simulink model "PassVeh7DOF"  (R2024b)
settings: Solver=ode14x  StartTime=0.0  StopTime=30  FixedStep=0.001  RelTol=1e-1
model workspace (MAT data in the model file):
  A_mu = 10
  B_reff = 8.386
  CONVERTER_DATA = [0 0.1 0.2 0.3 0.4 0.5 0.6 0.7 0.8 0.81 0.82 0.83 ... (63 elements, 21x3)]
  Cps = 2
  Cz = 7766.25
  DOWN_TABLE = [0 0 0 0 0 0 5 5 7.5 7.5 15 15 ... (30 elements, 6x5)]
  DOWN_TH_BP = [0 5 40 50 90 100]
  D_reff = 0.25826
  EMAP = [-40 215 245 264 264 267 267 267 267 267 -44 117 ... (110 elements, 10x11)]
  F0z = [6086.4 4324.8]
  F_reff = 0.07394
  F_zmax = 10000
  F_zmin = 100
  F_zo = 4000
  Kz = 48000
  MF : object (value not decoded)
  NCyl = 6
  NE_VEC = [800 1200 1600 2000 2400 2800 3200 3600 4000 4400 4800]
  Pstd = 101325
  R_eff = 0.298
  Rair = 287
  SUS : object (value not decoded)
  TH_VEC = [0; 20; 30; 40; 50; 60; 70; 80; 90; 100]
  TWAITdn = 1.25
  TWAITup = 0.1
  Tin = [1 2 3 4 5 6 7 8 9 10 2 2 ... (20 elements, 10x2)]
  Tstd = 293.15
  UP_TABLE = [7.5 7.5 15 25 40 40 25 25 35 45 70 80 ... (30 elements, 6x5)]
  UP_TH_BP = [0 25 35 50 90 100]
  VEH : object (value not decoded)
  V_o = 16.7
  V_xlow = 1
  Vd = 0.00346
  WH : object (value not decoded)
  a = 1.515
  alpha_max = 1.5
  alpha_min = -1.5
  b = 1.504
  c_zo = 209651
  epsilon = 0.1
  f_air = [0 0 0 0 0 0 0 0 0 0 0 0 ... (256 elements, 16x16)]
  f_co = [0 0 0 0 0 0 0 0 0 0 0 0 ... (256 elements, 16x16)]
  f_co2 = [0 0 0 0 0 0 0 0 0 0 0 0 ... (256 elements, 16x16)]
  f_eff = [352.135682859 352.135682859 320.724378192 303.655312657 295.930136708 291.240087194 291.240271258 291.240312459 291.240275452 291.240198499 291.240100781 291.240018769 ... (256 elements, 16x16)]
  f_fuel = [0 0 0 0 0 0 0 0 0 0 0 0 ... (256 elements, 16x16)]
  f_hc = [0 0 0 0 0 0 0 0 0 0 0 0 ... (256 elements, 16x16)]
  f_nox = [0 0 0 0 0 0 0 0 0 0 0 0 ... (256 elements, 16x16)]
  f_pm = [0 0 0 0 0 0 0 0 0 0 0 0 ... (256 elements, 16x16)]
  f_susp_axl_bp = [1 2]
  f_susp_dz_bp = [-4 -0.14 -0.13 -0.12 -0.11 -0.1 -0.09 -0.08 -0.07 -0.06 -0.05 -0.04 ... (31 elements, 1x31)]
  f_susp_dzdot_bp = [-4 -0.14 -0.13 -0.12 -0.11 -0.1 -0.09 -0.08 -0.07 -0.06 -0.05 -0.04 ... (31 elements, 1x31)]
  f_susp_fmz = [-213379.591456 -28099.591456 -27619.591456 -27139.591456 -26659.591456 -26179.591456 -25699.591456 -25219.591456 -24739.591456 -24259.591456 -23779.591456 -23299.591456 ... (468968 elements, 31x31x61x2x4)]
  f_susp_geom = [-0.832564012244 0.043269987756 0.045538987756 0.047807987756 0.050076987756 0.052345987756 0.054614987756 0.056883987756 0.059152987756 0.061421987756 0.063690987756 0.065959987756 ... (11346 elements, 31x61x2x3)]
  f_susp_strgdelta_bp = [-0.523598775598 -0.506145483078 -0.488692190558 -0.471238898038 -0.453785605519 -0.436332312999 -0.418879020479 -0.401425727959 -0.383972435439 -0.366519142919 -0.349065850399 -0.331612557879 ... (61 elements, 1x61)]
  f_tbrake = [0 76.8593923996 105.140482948 131.533638111 157.926793274 176.658631717 176.65727296 176.656856686 176.656879077 176.657093756 176.657404516 176.65772406 ... (256 elements, 16x16)]
  f_tbrake_n_bpt = [0 649.519052838 912.419621844 1175.32019085 1438.22075986 1701.12132886 1964.02189787 2226.92246687 2489.82303588 2752.72360489 3015.62417389 3278.5247429 ... (16 elements, 1x16)]
  f_tbrake_t_bpt = [0 34.6410161514 61.0341713143 87.4273264773 113.82048164 140.213636803 166.606791966 192.999947129 219.393102292 245.786257455 272.179412618 298.572567781 ... (16 elements, 1x16)]
  f_texh = [766.752464599 766.752464599 786.17542386 801.679939032 884.591982581 910.574397722 910.571871054 910.570774534 910.570601632 910.570821151 910.571247242 910.571639815 ... (256 elements, 16x16)]
  f_twc_eff_co = [0.17 0.25 0.45 0.99 0.99 0.99 0.99]
  f_twc_eff_hc = [0.21 0.375 0.75 0.98 0.98 0.98 0.98]
  f_twc_eff_lam = [0.909090909 0.944055944 0.979020979 1 1.013986014 1.048951049 1.083916084]
  f_twc_eff_nox = [0.98 0.98 0.98 0.97 0.05 0.02 0]
  h = 0.134
  k_z = 50
  kappa_max = 1.5
  kappa_min = -1.5
  lam_Cx = 1
  lam_Cy = 1
  lam_Cz = 1
  lam_Ex = 1
  lam_Ey = 1
  lam_F_zo = 1
  lam_Hx = 1
  lam_Hy = 1
  lam_Kxkappa = 1
  lam_Kyalpha = 1
  lam_Kygamma = 1
  lam_Kzgamma = 1
  lam_Mr = 1
  lam_Mx = 1
  lam_My = 1
  lam_S = 1
  lam_VMx = 1
  lam_Vx = 1
  lam_Vy = 1
  lam_Vykappa = 1
  lam_muV = 0
  lam_mux = 1
  lam_muy = 1
  lam_t = 1
  lam_xalpha = 1
  lam_ykappa = 1
  numWheel = 4
  p_Cx1 = 1.579
  p_Cy1 = 1.3332
  p_Dx1 = 1.0422
  p_Dx2 = -0.08285
  p_Dx3 = 0
  p_Dy1 = 0.8784
  p_Dy2 = -0.06445
  p_Dy3 = 0
  p_Ex1 = 0.11185
  p_Ex2 = 0.3127
  p_Ex3 = 0
  p_Ex4 = 0.001603
  p_Ey1 = -0.8227
  p_Ey2 = -0.6062
  p_Ey3 = 0.09825
  p_Ey4 = -6.546
  p_Ey5 = 0
  p_Fz1 = 0.7098
  p_Hx1 = 0.00021585
  p_Hx2 = 0.0011538
  p_Hy1 = -0.0018043
  p_Hy2 = 0.003518
  p_Kx1 = 21.69
  p_Kx2 = 13.774
  p_Kx3 = -0.4119
  p_Ky1 = -15.314
  p_Ky2 = 1.7044
  p_Ky3 = 0.36986
  p_Ky4 = 1.9896
  p_Ky5 = 0
  p_Ky6 = -0.9004
  p_Ky7 = -0.2328
  p_Vx1 = 1.5973e-05
  p_Vx2 = 0.0001043
  p_Vy1 = -0.006642
  p_Vy2 = 0.03597
  p_Vy3 = -0.1621
  p_Vy4 = -0.4908
  p_pmx1 = 0
  p_px1 = -0.3489
  p_px2 = 0.382
  p_px3 = -0.09634
  p_px4 = 0.06447
  p_py1 = -0.6249
  p_py2 = -0.06535
  p_py3 = -0.1668
  p_py4 = 0.2834
  p_py5 = 0
  path : object (value not decoded)
  pio = 220000
  q_Fcx = 0
  q_Fz2 = 15.4
  q_Fzy = 0
  q_reo = 0.9974
  q_sx1 = -0.007764
  q_sx10 = 0.2824
  q_sx11 = 5.349
  q_sx12 = 0
  q_sx13 = 0
  q_sx14 = 0
  q_sx2 = 1.1915
  q_sx3 = 0.013948
  q_sx4 = 4.912
  q_sx5 = 1.02
  q_sx6 = 22.83
  q_sx7 = 0.7104
  q_sx8 = -0.023393
  q_sx9 = 0.6581
  q_sy1 = 0.00702
  q_sy2 = 0
  q_sy3 = 0.001515
  q_sy4 = 8.514e-05
  q_sy5 = 0
  q_sy6 = 0
  q_sy7 = 0.9008
  q_sy8 = -0.4089
  q_v1 = 0.0007742
  q_v2 = 0.04667
  r_Bx1 = 12.531
  r_Bx2 = 9.532
  r_Bx3 = 0
  r_By1 = 10.615
  r_By2 = 7.705
  r_By3 = 3.433e-06
  r_By4 = 0
  r_Cx1 = 1.019
  r_Cy1 = 1.0585
  r_Ex1 = -0.4487
  r_Ex2 = -0.4726
  r_Ey1 = 0.3132
  r_Ey2 = 7.63e-06
  r_Hx1 = 0.0002374
  r_Hy1 = 0.011646
  r_Hy2 = 7.63e-06
  r_Vy1 = 0.05654
  r_Vy2 = 7.63e-06
  r_Vy3 = 0
  r_Vy4 = 99.9
  r_Vy5 = 2
  r_Vy6 = 15.814
  r_o = 0.3135
  reqTmaxT = [nan 0.285774810084 0.647179872268 nan nan nan nan nan nan nan nan nan ... (168 elements, 21x8)]
  vehSpd = [0 2.77777777778 5.55555555556 8.33333333333 11.1111111111 13.8888888889 16.6666666667 19.4444444444 22.2222222222 25 27.7777777778 30.5555555556 ... (21 elements, 1x21)]
  vehWidth = 2
  w = 1
symbols that are objects in the model workspace (value not decoded): VEH
undefined symbols (not defined in the file or in its folder): Fzz, Fzzdot, InertFrm, pFz, psi, vdyntiremask, x_o, zdotFz, zFz
libraries: simulink x4, sharedTrackingLibrary x1, mcbcontrolslib x1
(part 6 of 24)

== system PassVeh7DOF/Longitudinal Wheels 4DOF/Veh2Tire/Wheel to Body Transform ==
  VelVeh : Inport  Partition=on  PartitionDimension=2  PartitionWidth=1  PartitionOffset=0
  WhlAng : Inport  Port=2  Partition=on  PartitionDimension=2  PartitionWidth=1  PartitionOffset=0
  Demux1 : Demux  Outputs=3
  Divide1 : Product  Inputs=**  Multiplication=Matrix(*)
  For Each : ForEach  DisableCoverage=on
  Rotation Angles to Direction Cosine Matrix : Subsystem  mask(Ang2DCM){rotationOrder=ZYX, aMode=2}
      mask prompts: rotationOrder "shared_aeroblks:sharedaeroblktransform:blockAng2DCMParamRotationOrder"
      mask help: shared_aeroblks:sharedaeroblktransform:blockAng2DCMDesc
      mask init:
      | if aerosharedtest(gcb)
      |     ports=aerosharedicon('sharedang2dcm');
      | else
      |     ports=sharedautoicon('sharedang2dcm');
      | end
      settings: AttributesFormatString=Rotation Order: %<rotationOrder>
      mask Help: eval('if license(''test'',''Aerospace_Blockset'')aerosharedhelp(''rotation_angles_to_direction_cosine_matrix'');elseif license(''test'',''Powertrain_Blockset'')sharedautohelp(''rotation_angles_to_direction_cosine_matrix'');end')
      mask TypeOptions rotationOrder: shared_aeroblks:sharedaeroblktransform:blockParamComboZYX | shared_aeroblks:sharedaeroblktransform:blockParamComboZYZ | shared_aeroblks:sharedaeroblktransform:blockParamComboZXY | shared_aeroblks:sharedaeroblktransform:blockParamComboZXZ | shared_aeroblks:sharedaeroblktransform:blockParamComboYXZ | shared_aeroblks:sharedaeroblktransform:blockParamComboYXY | shared_aeroblks:sharedaeroblktransform:blockParamComboYZX | shared_aeroblks:sharedaeroblktransform:blockParamComboYZY | shared_aeroblks:sharedaeroblktransform:blockParamComboXYZ | shared_aeroblks:sharedaeroblktransform:blockParamComboXYX | shared_aeroblks:sharedaeroblktransform:blockParamComboXZY | shared_aeroblks:sharedaeroblktransform:blockParamComboXZX
      mask DialogControl rotationOrder Prompt: Rotation order:
      mask Display:
      | port_label('input',1,'[R_1,R_2,R_3]','texmode','on')
      | port_label('output',1,'DCM_{be}','texmode','on')
  Selector : Selector  InputPortWidth=3  IndexOptions=Index vector (dialog)  Indices=[3 2 1]  OutputSizes=1
  xdotWheel : Outport  ConcatenationDimension=1  VectorParamsAs1DForOutWhenUnconnected=off
  ydotWheel : Outport  Port=2  ConcatenationDimension=1  VectorParamsAs1DForOutWhenUnconnected=off
  zdotWheel : Outport  Port=3  ConcatenationDimension=1  VectorParamsAs1DForOutWhenUnconnected=off
  wires:
  Divide1/1 -> Demux1/1
  Demux1/1 -> xdotWheel/1
  Demux1/2 -> ydotWheel/1
  Demux1/3 -> zdotWheel/1
  Rotation Angles to Direction Cosine Matrix/1(Out1) -> Divide1/1
  VelVeh/1 -> Divide1/2
  WhlAng/1 -> Selector/1
  Selector/1 -> Rotation Angles to Direction Cosine Matrix/1(In1)

== system PassVeh7DOF/Longitudinal Wheels 4DOF/Velocity and Vertical Load/Bicycle ==
  VehFdbk : Inport
  Bicycle Fz : Subsystem
  Bicycle V : Subsystem
  VehVel : Outport  PortDimensions=[3,4]  VectorParamsAs1DForOutWhenUnconnected=off
  Fz : Outport  Port=2  VectorParamsAs1DForOutWhenUnconnected=off
  wires:
  VehFdbk/1 -> Bicycle V/1(In1), Bicycle Fz/1(VehFdbk)
  Bicycle V/1(Out1) -> VehVel/1
  Bicycle Fz/1(Out1) -> Fz/1

== system PassVeh7DOF/Longitudinal Wheels 4DOF/Velocity and Vertical Load/Dual ==
  VehFdbk : Inport
  Dual Fz : Subsystem
  Dual V : Subsystem
  VehVel : Outport  VectorParamsAs1DForOutWhenUnconnected=off
  Fz : Outport  Port=2  VectorParamsAs1DForOutWhenUnconnected=off
  wires:
  Dual V/1(Out1) -> VehVel/1
  VehFdbk/1 -> Dual Fz/1(In1), Dual V/1(In1)
  Dual Fz/1(Out1) -> Fz/1

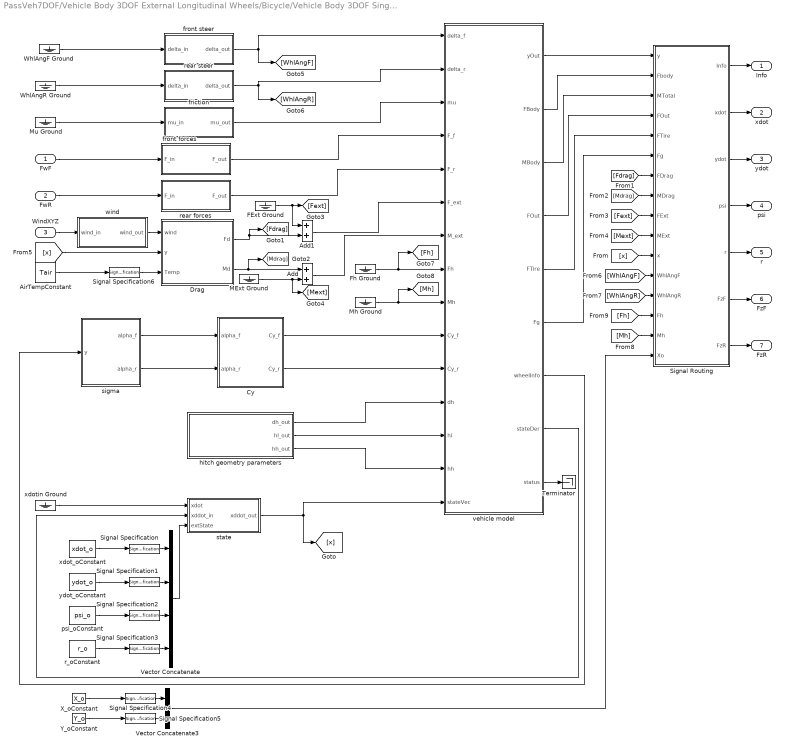
== system PassVeh7DOF/Vehicle Body 3DOF External Longitudinal Wheels/Bicycle/Vehicle Body 3DOF Single Track ==
  FwF : Inport
  FwR : Inport  Port=2
  WindXYZ : Inport  Port=3
  Add : Sum
  Add1 : Sum
  AirTempConstant : Constant  Value=Tair
  Cy : Subsystem  Variant=on  VariantControlMode=label  LabelModeActiveChoice=0
  Drag : Subsystem
  FExt Ground : Ground
  Fh Ground : Ground
  MExt Ground : Ground
  Mh Ground : Ground
  Mu Ground : Ground
  Signal Routing : Subsystem  Variant=on  VariantControlMode=label  LabelModeActiveChoice=0
  Signal Specification : SignalSpecification  Unit=m/s
  Signal Specification1 : SignalSpecification  Unit=m/s
  Signal Specification2 : SignalSpecification  Unit=rad
  Signal Specification3 : SignalSpecification  Unit=rad/s
  Signal Specification4 : SignalSpecification  Unit=m
  Signal Specification5 : SignalSpecification  Unit=m
  Signal Specification6 : SignalSpecification  Unit=K
  Terminator : Terminator
  Vector Concatenate : Concatenate  NumInputs=4
  Vector Concatenate3 : Concatenate
  WhlAngF Ground : Ground
  WhlAngR Ground : Ground
  X_oConstant : Constant  Value=X_o
  Y_oConstant : Constant  Value=Y_o
  friction : Subsystem  Variant=on  VariantControlMode=label  LabelModeActiveChoice=0
  front forces : Subsystem  Variant=on  VariantControlMode=label  LabelModeActiveChoice=2
  front steer : Subsystem  Variant=on  VariantControlMode=label  LabelModeActiveChoice=0
  hitch geometry parameters : Subsystem  Variant=on  VariantControlMode=label  LabelModeActiveChoice=3
  psi_oConstant : Constant  Value=psi_o
  r_oConstant : Constant  Value=r_o
  rear forces : Subsystem  Variant=on  VariantControlMode=label  LabelModeActiveChoice=2
  rear steer : Subsystem  Variant=on  VariantControlMode=label  LabelModeActiveChoice=0
  sigma : Subsystem  Variant=on  VariantControlMode=label  LabelModeActiveChoice=0
  state : Subsystem  Variant=on  VariantControlMode=label  LabelModeActiveChoice=0
  vehicle model : MATLAB Function  TreatAsAtomicUnit=on
  wind : Subsystem  Variant=on  VariantControlMode=label  LabelModeActiveChoice=1
  xdot_oConstant : Constant  Value=xdot_o
  xdotin Ground : Ground
  ydot_oConstant : Constant  Value=ydot_o
  Info : Outport  VectorParamsAs1DForOutWhenUnconnected=off
  xdot : Outport  Port=2  VectorParamsAs1DForOutWhenUnconnected=off
  ydot : Outport  Port=3  VectorParamsAs1DForOutWhenUnconnected=off
  psi : Outport  Port=4  VectorParamsAs1DForOutWhenUnconnected=off
  r : Outport  Port=5  VectorParamsAs1DForOutWhenUnconnected=off
  FzF : Outport  Port=6  VectorParamsAs1DForOutWhenUnconnected=off
  FzR : Outport  Port=7  VectorParamsAs1DForOutWhenUnconnected=off
  wires:
  AirTempConstant/1 -> Signal Specification6/1
  [Fh] -> Signal Routing/14(Fh)
  [Mh] -> Signal Routing/15(Mh)
  hitch geometry parameters/3(hh_out) -> vehicle model/14(hh)
  hitch geometry parameters/2(hl_out) -> vehicle model/13(hl)
  hitch geometry parameters/1(dh_out) -> vehicle model/12(dh)
  Mh Ground/1 -> [Mh], vehicle model/9(Mh)
  Fh Ground/1 -> [Fh], vehicle model/8(Fh)
  FExt Ground/1 -> [Fext], Add1/1
  MExt Ground/1 -> Add/2, [Mext]
  FwR/1 -> rear forces/1(F_in)
  FwF/1 -> front forces/1(F_in)
  xdotin Ground/1 -> state/1(xdot)
  Signal Specification6/1 -> Drag/3(Temp)
  Signal Specification5/1 -> Vector Concatenate3/2
  Y_oConstant/1 -> Signal Specification5/1
  Signal Specification4/1 -> Vector Concatenate3/1
  X_oConstant/1 -> Signal Specification4/1
  Vector Concatenate3/1 -> Signal Routing/16(Xo)
  Signal Specification2/1 -> Vector Concatenate/3
  Signal Specification3/1 -> Vector Concatenate/4
  psi_oConstant/1 -> Signal Specification2/1
  r_oConstant/1 -> Signal Specification3/1
  Signal Specification1/1 -> Vector Concatenate/2
  ydot_oConstant/1 -> Signal Specification1/1
  Signal Specification/1 -> Vector Concatenate/1
  xdot_oConstant/1 -> Signal Specification/1
  Vector Concatenate/1 -> state/3(extState)
  [WhlAngR] -> Signal Routing/13(WhlAngR)
  [WhlAngF] -> Signal Routing/12(WhlAngF)
  Signal Routing/4(psi) -> psi/1
  Mu Ground/1 -> friction/1(mu_in)
  WhlAngR Ground/1 -> rear steer/1(delta_in)
  [x] -> Drag/2(y)
  Drag/1(Fd) -> [Fdrag], Add1/2
  wind/1(wind_out) -> Drag/1(wind)
  Drag/2(Md) -> Add/1, [Mdrag]
  rear forces/1(F_out) -> vehicle model/5(F_r)
  front forces/1(F_out) -> vehicle model/4(F_f)
  vehicle model/7(wheelInfo) -> sigma/1(y)
  Signal Routing/1(Info) -> Info/1
  sigma/2(alpha_r) -> Cy/2(alpha_r)
  sigma/1(alpha_f) -> Cy/1(alpha_f)
  rear steer/1(delta_out) -> vehicle model/2(delta_r), [WhlAngR]
  front steer/1(delta_out) -> vehicle model/1(delta_f), [WhlAngF]
  Cy/2(Cy_r) -> vehicle model/11(Cy_r)
  Cy/1(Cy_f) -> vehicle model/10(Cy_f)
  friction/1(mu_out) -> vehicle model/3(mu)
  vehicle model/8(stateDer) -> state/2(xddot_in)
  vehicle model/1(yOut) -> Signal Routing/1(y)
  Signal Routing/3(ydot) -> ydot/1
  Signal Routing/5(r) -> r/1
  Signal Routing/6(FzF) -> FzF/1
  Signal Routing/7(FzR) -> FzR/1
  Signal Routing/2(xdot) -> xdot/1
  vehicle model/4(FOut) -> Signal Routing/4(FOut)
  state/1(xddot_out) -> vehicle model/15(stateVec), [x]
  [x] -> Signal Routing/11(x)
  vehicle model/9(status) -> Terminator/1
  vehicle model/5(FTire) -> Signal Routing/5(FTire)
  vehicle model/6(Fg) -> Signal Routing/6(Fg)
  [Fext] -> Signal Routing/9(FExt)
  [Fdrag] -> Signal Routing/7(FDrag)
  [Mdrag] -> Signal Routing/8(MDrag)
  [Mext] -> Signal Routing/10(MExt)
  vehicle model/2(FBody) -> Signal Routing/2(Fbody)
  vehicle model/3(MBody) -> Signal Routing/3(MTotal)
  Add/1 -> vehicle model/7(M_ext)
  Add1/1 -> vehicle model/6(F_ext)
  WhlAngF Ground/1 -> front steer/1(delta_in)
  WindXYZ/1 -> wind/1(wind_in)

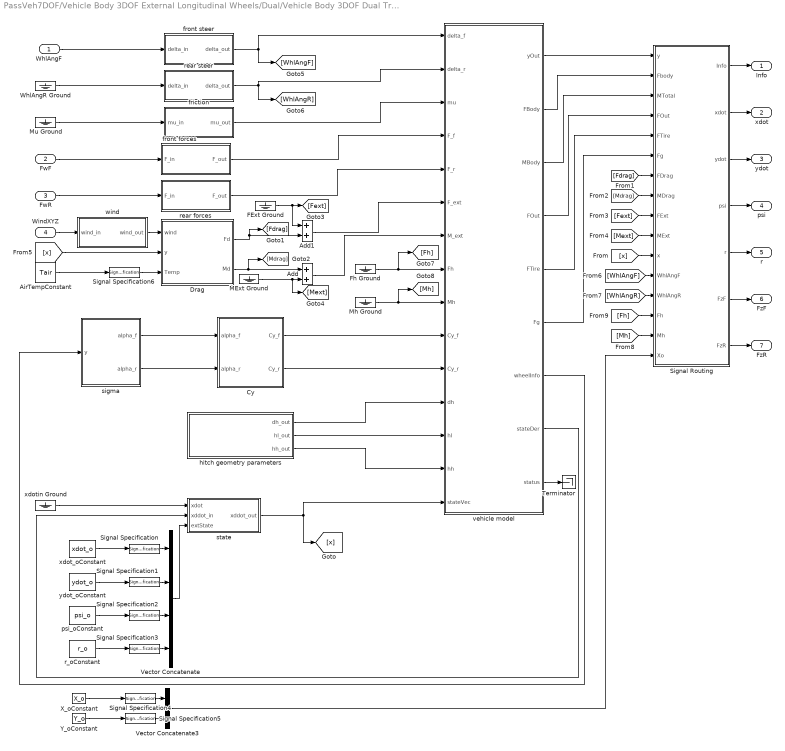
== system PassVeh7DOF/Vehicle Body 3DOF External Longitudinal Wheels/Dual/Vehicle Body 3DOF Dual Track ==
  WhlAngF : Inport
  FwF : Inport  Port=2
  FwR : Inport  Port=3
  WindXYZ : Inport  Port=4
  Add : Sum
  Add1 : Sum
  AirTempConstant : Constant  Value=Tair
  Cy : Subsystem  Variant=on  VariantControlMode=label  LabelModeActiveChoice=2
  Drag : Subsystem
  FExt Ground : Ground
  Fh Ground : Ground
  MExt Ground : Ground
  Mh Ground : Ground
  Mu Ground : Ground
  Signal Routing : Subsystem  Variant=on  VariantControlMode=label  LabelModeActiveChoice=1
  Signal Specification : SignalSpecification  Unit=m/s
  Signal Specification1 : SignalSpecification  Unit=m/s
  Signal Specification2 : SignalSpecification  Unit=rad
  Signal Specification3 : SignalSpecification  Unit=rad/s
  Signal Specification4 : SignalSpecification  Unit=m
  Signal Specification5 : SignalSpecification  Unit=m
  Signal Specification6 : SignalSpecification  Unit=K
  Terminator : Terminator
  Vector Concatenate : Concatenate  NumInputs=4
  Vector Concatenate3 : Concatenate
  WhlAngR Ground : Ground
  X_oConstant : Constant  Value=X_o
  Y_oConstant : Constant  Value=Y_o
  friction : Subsystem  Variant=on  VariantControlMode=label  LabelModeActiveChoice=2
  front forces : Subsystem  Variant=on  VariantControlMode=label  LabelModeActiveChoice=5
  front steer : Subsystem  Variant=on  VariantControlMode=label  LabelModeActiveChoice=3
  hitch geometry parameters : Subsystem  Variant=on  VariantControlMode=label  LabelModeActiveChoice=3
  psi_oConstant : Constant  Value=psi_o
  r_oConstant : Constant  Value=r_o
  rear forces : Subsystem  Variant=on  VariantControlMode=label  LabelModeActiveChoice=5
  rear steer : Subsystem  Variant=on  VariantControlMode=label  LabelModeActiveChoice=2
  sigma : Subsystem  Variant=on  VariantControlMode=label  LabelModeActiveChoice=2
  state : Subsystem  Variant=on  VariantControlMode=label  LabelModeActiveChoice=0
  vehicle model : MATLAB Function  TreatAsAtomicUnit=on
  wind : Subsystem  Variant=on  VariantControlMode=label  LabelModeActiveChoice=1
  xdot_oConstant : Constant  Value=xdot_o
  xdotin Ground : Ground
  ydot_oConstant : Constant  Value=ydot_o
  Info : Outport  VectorParamsAs1DForOutWhenUnconnected=off
  xdot : Outport  Port=2  VectorParamsAs1DForOutWhenUnconnected=off
  ydot : Outport  Port=3  VectorParamsAs1DForOutWhenUnconnected=off
  psi : Outport  Port=4  VectorParamsAs1DForOutWhenUnconnected=off
  r : Outport  Port=5  VectorParamsAs1DForOutWhenUnconnected=off
  FzF : Outport  Port=6  VectorParamsAs1DForOutWhenUnconnected=off
  FzR : Outport  Port=7  VectorParamsAs1DForOutWhenUnconnected=off
  wires:
  AirTempConstant/1 -> Signal Specification6/1
  [Fh] -> Signal Routing/14(Fh)
  [Mh] -> Signal Routing/15(Mh)
  hitch geometry parameters/3(hh_out) -> vehicle model/14(hh)
  hitch geometry parameters/2(hl_out) -> vehicle model/13(hl)
  hitch geometry parameters/1(dh_out) -> vehicle model/12(dh)
  Mh Ground/1 -> [Mh], vehicle model/9(Mh)
  Fh Ground/1 -> [Fh], vehicle model/8(Fh)
  FExt Ground/1 -> [Fext], Add1/1
  MExt Ground/1 -> Add/2, [Mext]
  FwR/1 -> rear forces/1(F_in)
  FwF/1 -> front forces/1(F_in)
  xdotin Ground/1 -> state/1(xdot)
  Signal Specification6/1 -> Drag/3(Temp)
  Signal Specification5/1 -> Vector Concatenate3/2
  Y_oConstant/1 -> Signal Specification5/1
  Signal Specification4/1 -> Vector Concatenate3/1
  X_oConstant/1 -> Signal Specification4/1
  Vector Concatenate3/1 -> Signal Routing/16(Xo)
  Signal Specification2/1 -> Vector Concatenate/3
  Signal Specification3/1 -> Vector Concatenate/4
  psi_oConstant/1 -> Signal Specification2/1
  r_oConstant/1 -> Signal Specification3/1
  Signal Specification1/1 -> Vector Concatenate/2
  ydot_oConstant/1 -> Signal Specification1/1
  Signal Specification/1 -> Vector Concatenate/1
  xdot_oConstant/1 -> Signal Specification/1
  Vector Concatenate/1 -> state/3(extState)
  [WhlAngR] -> Signal Routing/13(WhlAngR)
  [WhlAngF] -> Signal Routing/12(WhlAngF)
  Signal Routing/4(psi) -> psi/1
  Mu Ground/1 -> friction/1(mu_in)
  WhlAngR Ground/1 -> rear steer/1(delta_in)
  WhlAngF/1 -> front steer/1(delta_in)
  [x] -> Drag/2(y)
  Drag/1(Fd) -> [Fdrag], Add1/2
  wind/1(wind_out) -> Drag/1(wind)
  Drag/2(Md) -> Add/1, [Mdrag]
  rear forces/1(F_out) -> vehicle model/5(F_r)
  front forces/1(F_out) -> vehicle model/4(F_f)
  vehicle model/7(wheelInfo) -> sigma/1(y)
  Signal Routing/1(Info) -> Info/1
  sigma/2(alpha_r) -> Cy/2(alpha_r)
  sigma/1(alpha_f) -> Cy/1(alpha_f)
  rear steer/1(delta_out) -> vehicle model/2(delta_r), [WhlAngR]
  front steer/1(delta_out) -> vehicle model/1(delta_f), [WhlAngF]
  Cy/2(Cy_r) -> vehicle model/11(Cy_r)
  Cy/1(Cy_f) -> vehicle model/10(Cy_f)
  friction/1(mu_out) -> vehicle model/3(mu)
  vehicle model/8(stateDer) -> state/2(xddot_in)
  vehicle model/1(yOut) -> Signal Routing/1(y)
  Signal Routing/3(ydot) -> ydot/1
  Signal Routing/5(r) -> r/1
  Signal Routing/6(FzF) -> FzF/1
  Signal Routing/7(FzR) -> FzR/1
  Signal Routing/2(xdot) -> xdot/1
  vehicle model/4(FOut) -> Signal Routing/4(FOut)
  state/1(xddot_out) -> vehicle model/15(stateVec), [x]
  [x] -> Signal Routing/11(x)
  vehicle model/9(status) -> Terminator/1
  vehicle model/5(FTire) -> Signal Routing/5(FTire)
  vehicle model/6(Fg) -> Signal Routing/6(Fg)
  [Fext] -> Signal Routing/9(FExt)
  [Fdrag] -> Signal Routing/7(FDrag)
  [Mdrag] -> Signal Routing/8(MDrag)
  [Mext] -> Signal Routing/10(MExt)
  vehicle model/2(FBody) -> Signal Routing/2(Fbody)
  vehicle model/3(MBody) -> Signal Routing/3(MTotal)
  Add/1 -> vehicle model/7(M_ext)
  Add1/1 -> vehicle model/6(F_ext)
  WindXYZ/1 -> wind/1(wind_in)

== system PassVeh7DOF/Longitudinal Wheels 4DOF/Axle Forces/Bicycle/Wheel Angles ==
  Front : Inport
  Camber : Inport  Port=2
  Constant : Constant  Value=zeros(4,1)
  Reshape : Reshape  OutputDimensionality=Row vector (2-D)
  Reshape1 : Reshape  OutputDimensionality=Row vector (2-D)
  Reshape2 : Reshape  OutputDimensionality=Row vector (2-D)
  Vector Concatenate3 : Concatenate  NumInputs=3  Mode=Multidimensional array
  Vehicle : Outport  VectorParamsAs1DForOutWhenUnconnected=off
  wires:
  Reshape/1 -> Vector Concatenate3/3
  Reshape2/1 -> Vector Concatenate3/2
  Vector Concatenate3/1 -> Vehicle/1
  Reshape1/1 -> Vector Concatenate3/1
  Front/1 -> Reshape/1
  Camber/1 -> Reshape1/1
  Constant/1 -> Reshape2/1

== system PassVeh7DOF/Longitudinal Wheels 4DOF/Axle Forces/Bicycle/Wheel to Body Transform ==
  Forces : Inport  PortDimensions=[3,1]  Partition=on  PartitionDimension=2  PartitionWidth=1  PartitionOffset=0
  WheelAngles : Inport  Port=2  Partition=on  PartitionDimension=2  PartitionWidth=1  PartitionOffset=0
  Constant : Constant  Value=[pi;0;0]
  Demux1 : Demux  Outputs=3
  Divide1 : Product  Inputs=***  Multiplication=Matrix(*)
  For Each : ForEach  DisableCoverage=on
  Rotation Angles to Direction Cosine Matrix : Subsystem  mask(Ang2DCM){rotationOrder=ZYX, aMode=2}
      mask prompts: rotationOrder "shared_aeroblks:sharedaeroblktransform:blockAng2DCMParamRotationOrder"
      mask help: shared_aeroblks:sharedaeroblktransform:blockAng2DCMDesc
      mask init:
      | if aerosharedtest(gcb)
      |     ports=aerosharedicon('sharedang2dcm');
      | else
      |     ports=sharedautoicon('sharedang2dcm');
      | end
      settings: AttributesFormatString=Rotation Order: %<rotationOrder>
      mask Help: eval('if license(''test'',''Aerospace_Blockset'')aerosharedhelp(''rotation_angles_to_direction_cosine_matrix'');elseif license(''test'',''Powertrain_Blockset'')sharedautohelp(''rotation_angles_to_direction_cosine_matrix'');end')
      mask TypeOptions rotationOrder: shared_aeroblks:sharedaeroblktransform:blockParamComboZYX | shared_aeroblks:sharedaeroblktransform:blockParamComboZYZ | shared_aeroblks:sharedaeroblktransform:blockParamComboZXY | shared_aeroblks:sharedaeroblktransform:blockParamComboZXZ | shared_aeroblks:sharedaeroblktransform:blockParamComboYXZ | shared_aeroblks:sharedaeroblktransform:blockParamComboYXY | shared_aeroblks:sharedaeroblktransform:blockParamComboYZX | shared_aeroblks:sharedaeroblktransform:blockParamComboYZY | shared_aeroblks:sharedaeroblktransform:blockParamComboXYZ | shared_aeroblks:sharedaeroblktransform:blockParamComboXYX | shared_aeroblks:sharedaeroblktransform:blockParamComboXZY | shared_aeroblks:sharedaeroblktransform:blockParamComboXZX
      mask DialogControl rotationOrder Prompt: Rotation order:
      mask Display:
      | port_label('input',1,'[R_1,R_2,R_3]','texmode','on')
      | port_label('output',1,'DCM_{be}','texmode','on')
  Rotation Angles to Direction Cosine Matrix1 : Subsystem  mask(Ang2DCM){rotationOrder=ZYX, aMode=2}
      mask prompts: rotationOrder "shared_aeroblks:sharedaeroblktransform:blockAng2DCMParamRotationOrder"
      mask help: shared_aeroblks:sharedaeroblktransform:blockAng2DCMDesc
      mask init:
      | if aerosharedtest(gcb)
      |     ports=aerosharedicon('sharedang2dcm');
      | else
      |     ports=sharedautoicon('sharedang2dcm');
      | end
      settings: AttributesFormatString=Rotation Order: %<rotationOrder>
      mask Help: eval('if license(''test'',''Aerospace_Blockset'')aerosharedhelp(''rotation_angles_to_direction_cosine_matrix'');elseif license(''test'',''Powertrain_Blockset'')sharedautohelp(''rotation_angles_to_direction_cosine_matrix'');end')
      mask TypeOptions rotationOrder: shared_aeroblks:sharedaeroblktransform:blockParamComboZYX | shared_aeroblks:sharedaeroblktransform:blockParamComboZYZ | shared_aeroblks:sharedaeroblktransform:blockParamComboZXY | shared_aeroblks:sharedaeroblktransform:blockParamComboZXZ | shared_aeroblks:sharedaeroblktransform:blockParamComboYXZ | shared_aeroblks:sharedaeroblktransform:blockParamComboYXY | shared_aeroblks:sharedaeroblktransform:blockParamComboYZX | shared_aeroblks:sharedaeroblktransform:blockParamComboYZY | shared_aeroblks:sharedaeroblktransform:blockParamComboXYZ | shared_aeroblks:sharedaeroblktransform:blockParamComboXYX | shared_aeroblks:sharedaeroblktransform:blockParamComboXZY | shared_aeroblks:sharedaeroblktransform:blockParamComboXZX
      mask DialogControl rotationOrder Prompt: Rotation order:
      mask Display:
      | port_label('input',1,'[R_1,R_2,R_3]','texmode','on')
      | port_label('output',1,'DCM_{be}','texmode','on')
  Selector : Selector  InputPortWidth=3  IndexOptions=Index vector (dialog)  Indices=[3 2 1]  OutputSizes=1
  Selector1 : Selector  InputPortWidth=3  IndexOptions=Index vector (dialog)  Indices=[3 2 1]  OutputSizes=1
  Transpose : Math  Operator=transpose
  Fx : Outport  ConcatenationDimension=1  VectorParamsAs1DForOutWhenUnconnected=off
  Fy : Outport  Port=2  ConcatenationDimension=1  VectorParamsAs1DForOutWhenUnconnected=off
  Fz : Outport  Port=3  ConcatenationDimension=1  VectorParamsAs1DForOutWhenUnconnected=off
  wires:
  Demux1/1 -> Fx/1
  Demux1/2 -> Fy/1
  Demux1/3 -> Fz/1
  Rotation Angles to Direction Cosine Matrix/1(Out1) -> Transpose/1
  Forces/1 -> Divide1/3
  WheelAngles/1 -> Selector/1
  Selector/1 -> Rotation Angles to Direction Cosine Matrix/1(In1)
  Rotation Angles to Direction Cosine Matrix1/1(Out1) -> Divide1/2
  Divide1/1 -> Demux1/1
  Selector1/1 -> Rotation Angles to Direction Cosine Matrix1/1(In1)
  Constant/1 -> Selector1/1
  Transpose/1 -> Divide1/1

== system PassVeh7DOF/Longitudinal Wheels 4DOF/Axle Forces/Dual/Wheel Angles ==
  Front : Inport
  Camber : Inport  Port=2
  Constant : Constant  Value=zeros(4,1)
  Reshape : Reshape  OutputDimensionality=Row vector (2-D)
  Reshape1 : Reshape  OutputDimensionality=Row vector (2-D)
  Reshape2 : Reshape  OutputDimensionality=Row vector (2-D)
  Vector Concatenate3 : Concatenate  NumInputs=3  Mode=Multidimensional array
  Vehicle : Outport  VectorParamsAs1DForOutWhenUnconnected=off
  wires:
  Reshape/1 -> Vector Concatenate3/3
  Reshape2/1 -> Vector Concatenate3/2
  Vector Concatenate3/1 -> Vehicle/1
  Reshape1/1 -> Vector Concatenate3/1
  Front/1 -> Reshape/1
  Camber/1 -> Reshape1/1
  Constant/1 -> Reshape2/1

== system PassVeh7DOF/Longitudinal Wheels 4DOF/Axle Forces/Dual/Wheel to Body Transform ==
  Forces : Inport  PortDimensions=[3,1]  Partition=on  PartitionDimension=2  PartitionWidth=1  PartitionOffset=0
  WheelAngles : Inport  Port=2  Partition=on  PartitionDimension=2  PartitionWidth=1  PartitionOffset=0
  Constant : Constant  Value=[pi;0;0]
  Demux1 : Demux  Outputs=3
  Divide1 : Product  Inputs=***  Multiplication=Matrix(*)
  For Each : ForEach  DisableCoverage=on
  Rotation Angles to Direction Cosine Matrix : Subsystem  mask(Ang2DCM){rotationOrder=ZYX, aMode=2}
      mask prompts: rotationOrder "shared_aeroblks:sharedaeroblktransform:blockAng2DCMParamRotationOrder"
      mask help: shared_aeroblks:sharedaeroblktransform:blockAng2DCMDesc
      mask init:
      | if aerosharedtest(gcb)
      |     ports=aerosharedicon('sharedang2dcm');
      | else
      |     ports=sharedautoicon('sharedang2dcm');
      | end
      settings: AttributesFormatString=Rotation Order: %<rotationOrder>
      mask Help: eval('if license(''test'',''Aerospace_Blockset'')aerosharedhelp(''rotation_angles_to_direction_cosine_matrix'');elseif license(''test'',''Powertrain_Blockset'')sharedautohelp(''rotation_angles_to_direction_cosine_matrix'');end')
      mask TypeOptions rotationOrder: shared_aeroblks:sharedaeroblktransform:blockParamComboZYX | shared_aeroblks:sharedaeroblktransform:blockParamComboZYZ | shared_aeroblks:sharedaeroblktransform:blockParamComboZXY | shared_aeroblks:sharedaeroblktransform:blockParamComboZXZ | shared_aeroblks:sharedaeroblktransform:blockParamComboYXZ | shared_aeroblks:sharedaeroblktransform:blockParamComboYXY | shared_aeroblks:sharedaeroblktransform:blockParamComboYZX | shared_aeroblks:sharedaeroblktransform:blockParamComboYZY | shared_aeroblks:sharedaeroblktransform:blockParamComboXYZ | shared_aeroblks:sharedaeroblktransform:blockParamComboXYX | shared_aeroblks:sharedaeroblktransform:blockParamComboXZY | shared_aeroblks:sharedaeroblktransform:blockParamComboXZX
      mask DialogControl rotationOrder Prompt: Rotation order:
      mask Display:
      | port_label('input',1,'[R_1,R_2,R_3]','texmode','on')
      | port_label('output',1,'DCM_{be}','texmode','on')
  Rotation Angles to Direction Cosine Matrix1 : Subsystem  mask(Ang2DCM){rotationOrder=ZYX, aMode=2}
      mask prompts: rotationOrder "shared_aeroblks:sharedaeroblktransform:blockAng2DCMParamRotationOrder"
      mask help: shared_aeroblks:sharedaeroblktransform:blockAng2DCMDesc
      mask init:
      | if aerosharedtest(gcb)
      |     ports=aerosharedicon('sharedang2dcm');
      | else
      |     ports=sharedautoicon('sharedang2dcm');
      | end
      settings: AttributesFormatString=Rotation Order: %<rotationOrder>
      mask Help: eval('if license(''test'',''Aerospace_Blockset'')aerosharedhelp(''rotation_angles_to_direction_cosine_matrix'');elseif license(''test'',''Powertrain_Blockset'')sharedautohelp(''rotation_angles_to_direction_cosine_matrix'');end')
      mask TypeOptions rotationOrder: shared_aeroblks:sharedaeroblktransform:blockParamComboZYX | shared_aeroblks:sharedaeroblktransform:blockParamComboZYZ | shared_aeroblks:sharedaeroblktransform:blockParamComboZXY | shared_aeroblks:sharedaeroblktransform:blockParamComboZXZ | shared_aeroblks:sharedaeroblktransform:blockParamComboYXZ | shared_aeroblks:sharedaeroblktransform:blockParamComboYXY | shared_aeroblks:sharedaeroblktransform:blockParamComboYZX | shared_aeroblks:sharedaeroblktransform:blockParamComboYZY | shared_aeroblks:sharedaeroblktransform:blockParamComboXYZ | shared_aeroblks:sharedaeroblktransform:blockParamComboXYX | shared_aeroblks:sharedaeroblktransform:blockParamComboXZY | shared_aeroblks:sharedaeroblktransform:blockParamComboXZX
      mask DialogControl rotationOrder Prompt: Rotation order:
      mask Display:
      | port_label('input',1,'[R_1,R_2,R_3]','texmode','on')
      | port_label('output',1,'DCM_{be}','texmode','on')
  Selector : Selector  InputPortWidth=3  IndexOptions=Index vector (dialog)  Indices=[3 2 1]  OutputSizes=1
  Selector1 : Selector  InputPortWidth=3  IndexOptions=Index vector (dialog)  Indices=[3 2 1]  OutputSizes=1
  Transpose : Math  Operator=transpose
  Fx : Outport  ConcatenationDimension=1  VectorParamsAs1DForOutWhenUnconnected=off
  Fy : Outport  Port=2  ConcatenationDimension=1  VectorParamsAs1DForOutWhenUnconnected=off
  Fz : Outport  Port=3  ConcatenationDimension=1  VectorParamsAs1DForOutWhenUnconnected=off
  wires:
  Demux1/1 -> Fx/1
  Demux1/2 -> Fy/1
  Demux1/3 -> Fz/1
  Rotation Angles to Direction Cosine Matrix/1(Out1) -> Transpose/1
  Forces/1 -> Divide1/3
  WheelAngles/1 -> Selector/1
  Selector/1 -> Rotation Angles to Direction Cosine Matrix/1(In1)
  Rotation Angles to Direction Cosine Matrix1/1(Out1) -> Divide1/2
  Divide1/1 -> Demux1/1
  Selector1/1 -> Rotation Angles to Direction Cosine Matrix1/1(In1)
  Constant/1 -> Selector1/1
  Transpose/1 -> Divide1/1

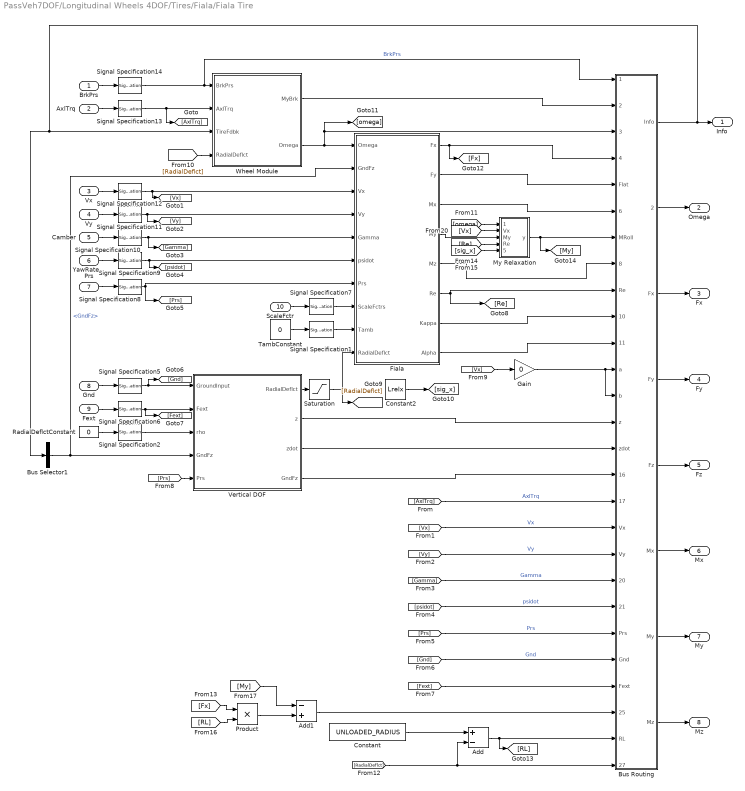
== system PassVeh7DOF/Longitudinal Wheels 4DOF/Tires/Fiala/Fiala Tire ==
  BrkPrs : Inport
  AxlTrq : Inport  Port=2
  Vx : Inport  Port=3
  Vy : Inport  Port=4
  Camber : Inport  Port=5
  YawRate : Inport  Port=6
  Prs : Inport  Port=7
  Gnd : Inport  Port=8
  Fext : Inport  Port=9
  ScaleFctr : Inport  Port=10
  Add : Sum  Inputs=+-
  Add1 : Sum  Inputs=-+
  Bus Selector1 : BusSelector  OutputSignals=GndFz
  Bus Routing : Subsystem
  Constant : Constant  Value=UNLOADED_RADIUS
  Constant2 : Constant  Value=Lrelx
  Fiala : Subsystem
  Gain : Gain  Gain=0
  My Relaxation : Subsystem
  Product : Product
  RadialDeflctConstant : Constant  Value=0
  Saturation : Saturate  UpperLimit=inf  LowerLimit=0
  Signal Specification1 : SignalSpecification  Unit=K
  Signal Specification10 : SignalSpecification  Unit=rad
  Signal Specification11 : SignalSpecification  Unit=m/s
  Signal Specification12 : SignalSpecification  Unit=m/s
  Signal Specification13 : SignalSpecification  Unit=N*m
  Signal Specification14 : SignalSpecification  Unit=Pa
  Signal Specification2 : SignalSpecification  Unit=m
  Signal Specification5 : SignalSpecification  Unit=m
  Signal Specification6 : SignalSpecification  Unit=N
  Signal Specification7 : SignalSpecification  Unit=1
  Signal Specification8 : SignalSpecification  Unit=Pa
  Signal Specification9 : SignalSpecification  Unit=rad/s
  TambConstant : Constant  Value=0
  Vertical DOF : Subsystem  Variant=on  VariantControl=Variant1
  Wheel Module : Subsystem  mask{Iyy=IYY}
      mask prompts: Iyy "Rotational inertia, Iyy [kg*m^2]:"
  Info : Outport  VectorParamsAs1DForOutWhenUnconnected=off
  Omega : Outport  Port=2  Unit=rad/s  VectorParamsAs1DForOutWhenUnconnected=off
  Fx : Outport  Port=3  Unit=N  VectorParamsAs1DForOutWhenUnconnected=off
  Fy : Outport  Port=4  Unit=N  VectorParamsAs1DForOutWhenUnconnected=off
  Fz : Outport  Port=5  Unit=N  VectorParamsAs1DForOutWhenUnconnected=off
  Mx : Outport  Port=6  Unit=N*m  VectorParamsAs1DForOutWhenUnconnected=off
  My : Outport  Port=7  Unit=N*m  VectorParamsAs1DForOutWhenUnconnected=off
  Mz : Outport  Port=8  Unit=N*m  VectorParamsAs1DForOutWhenUnconnected=off
  wires:
  RadialDeflctConstant/1 -> Signal Specification2/1
  Fext/1 -> Signal Specification6/1
  Saturation/1 -> Fiala/10(RadialDeflct), [RadialDeflct]
  Vertical DOF/1(RadialDeflct) -> Saturation/1
  [RadialDeflct] -> Bus Routing/27(RadialDeflct), Add/2
  [RL] -> Product/2
  Product/1 -> Add1/2
  [My] -> Add1/1
  Add1/1 -> Bus Routing/25(WhlTrq)
  [Fx] -> Product/1
  Add/1 -> Bus Routing/26(RL), [RL]
  Constant/1 -> Add/1
  BrkPrs/1 -> Signal Specification14/1
  Signal Specification2/1 -> Vertical DOF/3(rho)
  Constant2/1 -> [sig_x]
  Fiala/6(Re) -> [Re], Bus Routing/9(Re)
  [Re] -> My Relaxation/4(Re)
  [omega] -> My Relaxation/1(Omega)
  [Vx] -> My Relaxation/2(Vx)
  [sig_x] -> My Relaxation/5(sig_x)
  Wheel Module/1(MyBrk) -> Bus Routing/2(BrkTrq)
  Signal Specification5/1 -> Vertical DOF/1("GroundInput "), [Gnd]
  Gnd/1 -> Signal Specification5/1
  Signal Specification6/1 -> [Fext], Vertical DOF/2("Fext ")
  Signal Specification7/1 -> Fiala/8(ScaleFctrs)
  Prs/1 -> Signal Specification8/1
  Signal Specification8/1 -> [Prs], Fiala/7(Prs)
  YawRate/1 -> Signal Specification9/1
  Signal Specification9/1 -> [psidot], Fiala/6(psidot)
  ScaleFctr/1 -> Signal Specification7/1
  Signal Specification10/1 -> [Gamma], Fiala/5(Gamma)
  Camber/1 -> Signal Specification10/1
  Signal Specification11/1 -> [Vy], Fiala/4(Vy)
  Vy/1 -> Signal Specification11/1
  Vx/1 -> Signal Specification12/1
  Signal Specification12/1 -> [Vx], Fiala/3(Vx)
  Signal Specification13/1 -> [AxlTrq], Wheel Module/2(AxlTrq)
  AxlTrq/1 -> Signal Specification13/1
  Signal Specification14/1 -> Bus Routing/1(BrkPrs), Wheel Module/1(BrkPrs)  "BrkPrs"
  Bus Selector1/1 -> Vertical DOF/4("GndFz "), Fiala/2(GndFz)  "<GndFz>"
  Bus Routing/1(Info) -> Info/1, Wheel Module/3(TireFdbk), Bus Selector1/1
  Fiala/5(Mz) -> Bus Routing/8(MAlign)
  Fiala/7(Kappa) -> Bus Routing/10(Kappa)
  Fiala/8(Alpha) -> Bus Routing/11(Alpha)
  Bus Routing/2(Omega) -> Omega/1
  Bus Routing/3(Fx) -> Fx/1
  Bus Routing/4(Fy) -> Fy/1
  Bus Routing/5(Fz) -> Fz/1
  Bus Routing/6(Mx) -> Mx/1
  Bus Routing/7(My) -> My/1
  Bus Routing/8(Mz) -> Mz/1
  [AxlTrq] -> Bus Routing/17(AxlTrq)  "AxlTrq"
  [Vx] -> Bus Routing/18(Vx)  "Vx"
  [Vy] -> Bus Routing/19(Vy)  "Vy"
  [Gamma] -> Bus Routing/20(Gamma)  "Gamma"
  [psidot] -> Bus Routing/21(psidot)  "psidot"
  [Prs] -> Bus Routing/22(Prs)  "Prs"
  [Gnd] -> Bus Routing/23(Gnd)  "Gnd"
  [Fext] -> Bus Routing/24(Fext)
  Fiala/3(Mx) -> Bus Routing/6(MOver)
  Fiala/2(Fy) -> Bus Routing/5(Flat)
  Fiala/1(Fx) -> Bus Routing/4(FLong), [Fx]
  Fiala/4(My) -> My Relaxation/3(My)
  My Relaxation/1(y) -> Bus Routing/7(MRoll), [My]
  [RadialDeflct] -> Wheel Module/4(RadialDeflct)
  Signal Specification1/1 -> Fiala/9(Tamb)
  Vertical DOF/2(" z") -> Bus Routing/14(z)
  [Prs] -> Vertical DOF/5(Prs)
  TambConstant/1 -> Signal Specification1/1
  Vertical DOF/4(GndFz) -> Bus Routing/16(GndFz)
  Wheel Module/2(Omega) -> Bus Routing/3(omega), [omega], Fiala/1(Omega)
  Vertical DOF/3(" zdot") -> Bus Routing/15(zdot)
  [Vx] -> Gain/1
  Gain/1 -> Bus Routing/12(a), Bus Routing/13(b)

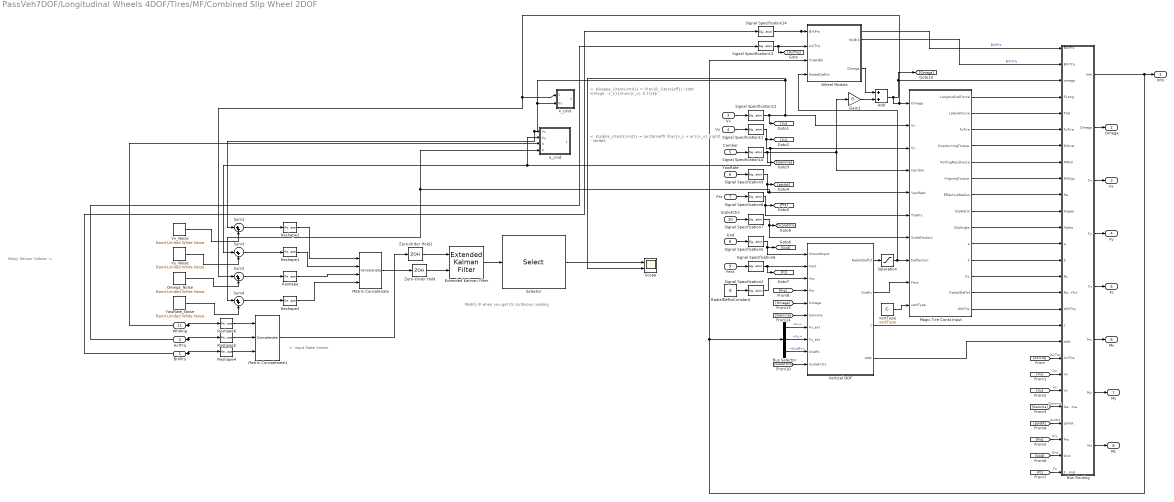
== system PassVeh7DOF/Longitudinal Wheels 4DOF/Tires/MF/Combined Slip Wheel 2DOF ==
  note: Modify B when you get its continous reading
  note: <- input State Vector
  note: Noisy Sensor Values
      | ->
  note: <- $\alpha_{\text{cmd}} = \arctan\left( \frac{v_y + ar}{v_x} \right) - \delta$
  note: <- $\kappa_{\text{cmd}} = \frac{R_{\text{eff}} \cdot \omega - v_x}{\max(|v_x|, 0.1)}$$
  BrkPrs : Inport
  AxlTrq : Inport  Port=2
  Vx : Inport  Port=3
  Vy : Inport  Port=4
  Camber : Inport  Port=5
  YawRate : Inport  Port=6
  Prs : Inport  Port=7
  Gnd : Inport  Port=8
  Fext : Inport  Port=9
  ScaleFctrs : Inport  Port=10
  WhlAng : Inport  Port=11
  Add : Sum
  Bus Selector : BusSelector  OutputSignals=Fx,Fy,GndFz
  Bus Routing : Subsystem
  Extended Kalman Filter : sharedTrackingLibrary/Extended Kalman Filter  StateTransitionFcn=myStateTransitionFcn  HasStateTransitionJacobianFcn=off  HasAdditiveProcessNoise=Additive  ProcessNoise=eye(16) * 1e-6  HasTimeVaryingProcessNoise=off  HasStateTransitionFcnExtraArgument=1  InitialState=zeros(16,1)  InitialStateCovariance=eye(16) * 0.01  MeasurementFcn1=myMeasurementFcn  HasMeasurementJacobianFcn1=off  HasMeasurementEnablePort1=off  HasAdditiveMeasurementNoise1=Additive  MeasurementNoise1=eye(16) * 0.1  HasTimeVaryingMeasurementNoise1=off  HasMeasurementFcnExtraArgument1=0  HasMeasurementWrapping1=off  MeasurementFcn2=myMeasurementFcn  HasMeasurementJacobianFcn2=off  HasMeasurementEnablePort2=off  HasAdditiveMeasurementNoise2=Additive  MeasurementNoise2=1  HasTimeVaryingMeasurementNoise2=off  HasMeasurementFcnExtraArgument2=0  HasMeasurementWrapping2=off  MeasurementFcn3=myMeasurementFcn  HasMeasurementJacobianFcn3=off  HasMeasurementEnablePort3=off  HasAdditiveMeasurementNoise3=Additive  MeasurementNoise3=1  HasTimeVaryingMeasurementNoise3=off  HasMeasurementFcnExtraArgument3=0  HasMeasurementWrapping3=off  MeasurementFcn4=myMeasurementFcn  HasMeasurementJacobianFcn4=off  HasMeasurementEnablePort4=off  HasAdditiveMeasurementNoise4=Additive  MeasurementNoise4=1  HasTimeVaryingMeasurementNoise4=off  HasMeasurementFcnExtraArgument4=0  HasMeasurementWrapping4=off  MeasurementFcn5=myMeasurementFcn  HasMeasurementJacobianFcn5=off  HasMeasurementEnablePort5=off  HasAdditiveMeasurementNoise5=Additive  MeasurementNoise5=1  HasTimeVaryingMeasurementNoise5=off  HasMeasurementFcnExtraArgument5=0  HasMeasurementWrapping5=off  EnableMultirate=off  StateTransitionFcnSampleTime=1  MeasurementFcn1SampleTime=1  MeasurementFcn2SampleTime=1  MeasurementFcn3SampleTime=1  MeasurementFcn4SampleTime=1  MeasurementFcn5SampleTime=1  UseCurrentEstimator=on  OutputStateCovariance=off  DataType=double  SampleTime=0.001  NumberOfMeasurements=1
  Gain1 : Gain  Gain=0
  Magic Tire Const Input : Subsystem
  Matrix Concatenate : Concatenate  NumInputs=4  Mode=Multidimensional array
  Matrix Concatenate1 : Concatenate  NumInputs=3  Mode=Multidimensional array
  Omega_Noise : simulink/Sources/Band-Limited White Noise  Cov=[0.0025]  Ts=0.01  seed=[23341]
  RadialDeflctConstant : Constant  Value=0
  Reshape{,1..6} (7 alike) : Reshape  OutputDimensionality=Column vector (2-D)
  Saturation : Saturate  UpperLimit=inf  LowerLimit=0
  Scope : Scope  NumInputPorts=2
  Selector : Selector  InputPortWidth=16  IndexOptions=Index vector (dialog)  Indices=1:4  OutputSizes=1
  Signal Specification10 : SignalSpecification  Unit=rad
  Signal Specification11 : SignalSpecification  Unit=m/s
  Signal Specification12 : SignalSpecification  Unit=m/s
  Signal Specification13 : SignalSpecification  Unit=N*m
  Signal Specification14 : SignalSpecification  Unit=Pa
  Signal Specification2 : SignalSpecification  Unit=m
  Signal Specification5 : SignalSpecification  Unit=m
  Signal Specification6 : SignalSpecification  Unit=N
  Signal Specification7 : SignalSpecification  Unit=1
  Signal Specification8 : SignalSpecification  Unit=Pa
  Signal Specification9 : SignalSpecification  Unit=rad/s
  Sum{1..4} (4 alike) : Sum  Inputs=|++
  Vertical DOF : Subsystem  Variant=on  VariantControl=Variant1
  Vx_Noise : simulink/Sources/Band-Limited White Noise  Cov=[0.0025]  Ts=0.01  seed=[23341]
  Vy_Noise : simulink/Sources/Band-Limited White Noise  Cov=[0.0004]  Ts=0.01  seed=[23341]
  Wheel Module : Subsystem  mask{Iyy=IYY}
      mask prompts: Iyy "Rotational inertia, Iyy [kg*m^2]:"
  YawRate_Noise : simulink/Sources/Band-Limited White Noise  Cov=[5*10^-5]  Ts=0.01  seed=[23341]
  Zero-Order Hold : ZeroOrderHold  SampleTime=0.001
  Zero-Order Hold1 : ZeroOrderHold  SampleTime=0.001
  a_cmd : Subsystem
  k_cmd : Subsystem
  vertType : Constant  Value=vertType
  Info : Outport  VectorParamsAs1DForOutWhenUnconnected=off
  Omega : Outport  Port=2  Unit=rad/s  VectorParamsAs1DForOutWhenUnconnected=off
  Fx : Outport  Port=3  Unit=N  VectorParamsAs1DForOutWhenUnconnected=off
  Fy : Outport  Port=4  Unit=N  VectorParamsAs1DForOutWhenUnconnected=off
  Fz : Outport  Port=5  Unit=N  VectorParamsAs1DForOutWhenUnconnected=off
  Mx : Outport  Port=6  Unit=N*m  VectorParamsAs1DForOutWhenUnconnected=off
  My : Outport  Port=7  Unit=N*m  VectorParamsAs1DForOutWhenUnconnected=off
  Mz : Outport  Port=8  Unit=N*m  VectorParamsAs1DForOutWhenUnconnected=off
  wires:
  RadialDeflctConstant/1 -> Signal Specification2/1
  Fext/1 -> Signal Specification6/1
  Saturation/1 -> Magic Tire Const Input/8(Deflection), Wheel Module/4(RadialDeflct)
  Vertical DOF/1(" RadialDeflct") -> Saturation/1
  Magic Tire Const Input/12(RL) -> Bus Routing/15(RL)
  Magic Tire Const Input/13(RadialDeflct) -> Bus Routing/16(RadialDeflct)
  Magic Tire Const Input/14(WhlTrq) -> Bus Routing/17(WhlTrq)
  Gain1/1 -> Add/2
  Wheel Module/2(Omega) -> Add/1
  Signal Specification2/1 -> Vertical DOF/3(rho)
  BrkPrs/1 -> Signal Specification14/1, Reshape4/1
  vertType/1 -> Magic Tire Const Input/10(vertType)
  Bus Selector/3 -> Vertical DOF/9("GndFz ")  "<GndFz>"
  [ScaleFctrs] -> Vertical DOF/10(ScaleFctrs)
  [Gamma] -> Vertical DOF/6(Gamma)
  [Omega] -> Vertical DOF/5(Omega)
  Bus Selector/1 -> Vertical DOF/7(Fx_ext)  "<Fx>"
  Bus Selector/2 -> Vertical DOF/8(Fy_ext)  "<Fy>"
  Magic Tire Const Input/3(FzTire) -> Bus Routing/6(FzTire)
  Vertical DOF/2(GndFz) -> Magic Tire Const Input/9(Fext)
  [Prs] -> Vertical DOF/4(Prs)
  [Fz] -> Bus Routing/27(FNormal)  "Fz"
  [Gnd] -> Bus Routing/26(Gnd)  "Gnd"
  [Prs] -> Bus Routing/25(Prs)  "Prs"
  [psidot] -> Bus Routing/24(psidot)  "psidot"
  [Gamma] -> Bus Routing/23(Gamma)  "Gamma"
  [Vy] -> Bus Routing/22(Vy)  "Vy"
  [Vx] -> Bus Routing/21(Vx)  "Vx"
  [AxlTrq] -> Bus Routing/20(AxlTrq)  "AxlTrq"
  Bus Routing/8(Mz) -> Mz/1
  Bus Routing/7(My) -> My/1
  Bus Routing/6(Mx) -> Mx/1
  Bus Routing/5(Fz) -> Fz/1
  Bus Routing/4(Fy) -> Fy/1
  Bus Routing/3(Fx) -> Fx/1
  Bus Routing/2(Omega) -> Omega/1
  Vertical DOF/4(" zdot") -> Bus Routing/19(zdot)
  Vertical DOF/3(" z") -> Bus Routing/18(z)
  Magic Tire Const Input/11(b) -> Bus Routing/14(b)
  Magic Tire Const Input/10(a) -> Bus Routing/13(a)
  Magic Tire Const Input/9(SlipAngle) -> Bus Routing/12(Alpha)
  Magic Tire Const Input/8(SlipRatio) -> Bus Routing/11(Kappa)
  Magic Tire Const Input/7(EffectiveRadius) -> Bus Routing/10(Re)
  Magic Tire Const Input/6(AligningTorque) -> Bus Routing/9(MAlign)
  Magic Tire Const Input/5(RollingResistance) -> Bus Routing/8(MRoll)
  Magic Tire Const Input/4(OverturningTorque) -> Bus Routing/7(MOver)
  Magic Tire Const Input/2(LateralForce) -> Bus Routing/5(Flat)
  Magic Tire Const Input/1(LongitudinalForce) -> Bus Routing/4(FLong)
  Bus Routing/1(Info) -> Bus Selector/1, Wheel Module/3(TireFdbk), Info/1
  Signal Specification14/1 -> Wheel Module/1(BrkPrs), Bus Routing/1(BrkPrs)  "BrkPrs"
  AxlTrq/1 -> Signal Specification13/1, Reshape5/1
  Signal Specification13/1 -> Wheel Module/2(AxlTrq), [AxlTrq]
  Signal Specification12/1 -> Magic Tire Const Input/2(Vx), Scope/2, Sum1/1, a_cmd/1(Vx), k_cmd/2(Vx), [Vx]
  Vx/1 -> Signal Specification12/1
  Vy/1 -> Signal Specification11/1
  Signal Specification11/1 -> Magic Tire Const Input/3(Vy), Sum3/1, a_cmd/2(Vy), [Vy]
  Camber/1 -> Signal Specification10/1
  Signal Specification10/1 -> Magic Tire Const Input/4(Camber), Gain1/1, [Gamma]
  ScaleFctrs/1 -> Signal Specification7/1
  Signal Specification9/1 -> Sum4/1, a_cmd/4(YawRate), Magic Tire Const Input/5(YawRate), [psidot]
  YawRate/1 -> Signal Specification9/1
  Signal Specification8/1 -> Magic Tire Const Input/6(TirePrs), [Prs]
  Prs/1 -> Signal Specification8/1
  Signal Specification7/1 -> Magic Tire Const Input/7(ScaleFactors), [ScaleFctrs]
  Signal Specification6/1 -> Vertical DOF/2("Fext "), [Fz]
  Gnd/1 -> Signal Specification5/1
  Signal Specification5/1 -> Vertical DOF/1("GroundInput "), [Gnd]
  Add/1 -> [Omega], Bus Routing/3(omega), Sum2/1, k_cmd/1(Omega), Magic Tire Const Input/1(Omega)
  Wheel Module/1(MyBrk) -> Bus Routing/2(BrkTrq)  "BrkTrq"
  WhlAng/1 -> Reshape6/1, a_cmd/3(WhlAng)
  Vx_Noise/1 -> Sum1/2
  Vy_Noise/1 -> Sum3/2
  Omega_Noise/1 -> Sum2/2
  YawRate_Noise/1 -> Sum4/2
  Matrix Concatenate1/1 -> Zero-Order Hold1/1
  Sum1/1 -> Reshape2/1
  Sum3/1 -> Reshape1/1
  Sum2/1 -> Reshape/1
  Sum4/1 -> Reshape3/1
  Matrix Concatenate/1 -> Zero-Order Hold/1
  Reshape/1 -> Matrix Concatenate/3
  Zero-Order Hold/1 -> Extended Kalman Filter/2
  Zero-Order Hold1/1 -> Extended Kalman Filter/1
  Extended Kalman Filter/1 -> Selector/1
  Reshape1/1 -> Matrix Concatenate/2
  Reshape2/1 -> Matrix Concatenate/1
  Reshape3/1 -> Matrix Concatenate/4
  Reshape4/1 -> Matrix Concatenate1/3
  Reshape5/1 -> Matrix Concatenate1/2
  Reshape6/1 -> Matrix Concatenate1/1
  Selector/1 -> Scope/1

== system PassVeh7DOF/Longitudinal Wheels 4DOF/Tires/MF/scale factors with friction ==
  lamda_mu_x : Inport
  lamda_mu_y : Inport  Port=2
  0 : Constant  Value=[zeros(1,numWheels)]  VectorParams1D=off
  Reshape : Reshape  OutputDimensionality=Row vector (2-D)  OutputDimensions=[1,numWheels]
  Reshape1 : Reshape  OutputDimensionality=Row vector (2-D)  OutputDimensions=[1,numWheels]
  Signal Specification3 : SignalSpecification  Unit=1
  Vector Concatenate : Concatenate  NumInputs=5  Mode=Multidimensional array
  ones : Constant  Value=[ones(23,numWheels)]  VectorParams1D=off
  ones2 : Constant  Value=ones(1,numWheels)  VectorParams1D=off
  lambdas : Outport  Unit=1  VectorParamsAs1DForOutWhenUnconnected=off
  wires:
  lamda_mu_y/1 -> Reshape1/1
  lamda_mu_x/1 -> Reshape/1
  ones2/1 -> Vector Concatenate/1  "lambda_Fz0"
  Vector Concatenate/1 -> Signal Specification3/1
  ones/1 -> Vector Concatenate/5
  0/1 -> Vector Concatenate/4  "lamda_mu_V"
  Reshape1/1 -> Vector Concatenate/3
  Reshape/1 -> Vector Concatenate/2
  Signal Specification3/1 -> lambdas/1
